simulink model "k1vissrmp_20190617"  (Simulink 8.6)
settings: Solver=ode45  StartTime=0.0  StopTime=10.0  RelTol=1e-3
libraries: cdsIPCx x5, cdsCDI64 x3, cdsCDO64 x3, TYPEB_MASTER x3, dac x2, cdsAdcx0 x1, cdsParameters x1
settings Model: Creator=controls  LastModifiedBy=controls
settings DataIOCC: SignalLoggingSaveFormat=Dataset
settings OptimizationCC: ExpressionDepthLimit=128
settings DebuggingCC: UnderspecifiedInitializationDetection=Simplified  MergeDetectMultiDrivingBlocksExec=error  SolverPrmCheckMsg=none  FcnCallInpInsideContextMsg=EnableAllAsError  StateNameClashWarn=none
settings GRTTargetCC: CombineOutputUpdateFcns=on  GRTInterface=off

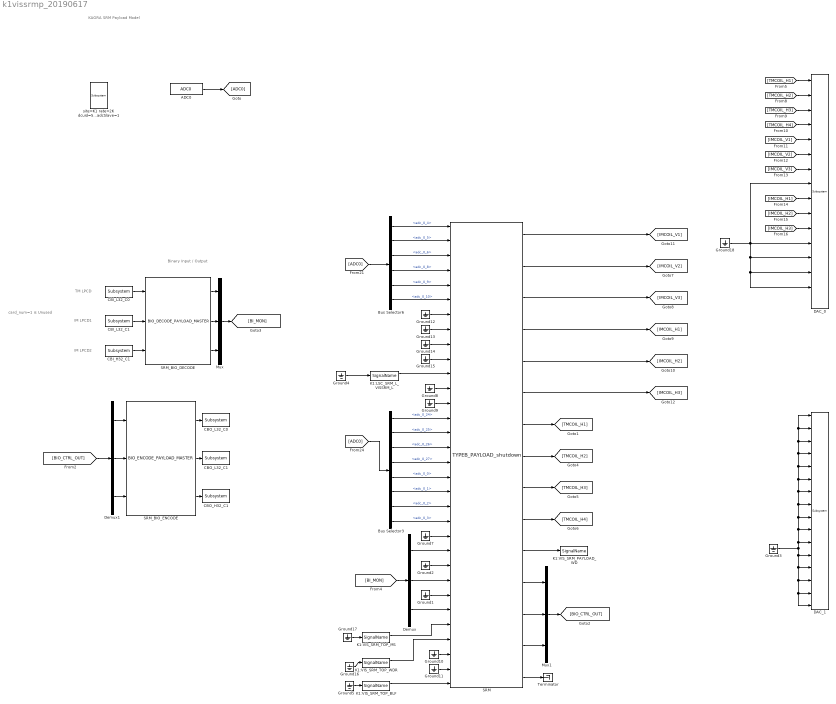
== system k1vissrmp_20190617 ==
  note: KAGRA SRM Payload Model
  note: Binary Input / Output
  note: TM LPCD
  note: card_num=1 is Unused
  note: IM LPCD1
  note: IM LPCD2
  ADC0 : cdsAdcx0/ADC0  Tag=cdsAdc  Description=|
      | type-GSC_16AI64SSA
      | card_num=0
      settings: AttributesFormatString=%<Description>\n%<Tag>
  Bus Selector3 : BusSelector  Description=ADC Selector  OutputSignals=adc_0_24,adc_0_25,adc_0_26,adc_0_27,adc_0_0,adc_0_1,adc_0_2,adc_0_3
      settings: AttributesFormatString=%<Description>
  Bus Selector6 : BusSelector  Description=ADC Selector  OutputSignals=adc_0_4,adc_0_5,adc_0_6,adc_0_8,adc_0_9,adc_0_10
      settings: AttributesFormatString=%<Description>
  CBI_H32_C1 : cdsCDI64/Subsystem  Tag=cdsCDI64  Description=card_num=3
      settings: AttributesFormatString=%<Tag>\n%<Description>
  CBI_L32_C0 : cdsCDI64/Subsystem  Tag=cdsCDI64  Description=card_num=0
      settings: AttributesFormatString=%<Tag>\n%<Description>
  CBI_L32_C1 : cdsCDI64/Subsystem  Tag=cdsCDI64  Description=card_num=2
      settings: AttributesFormatString=%<Tag>\n%<Description>
  CBO_H32_C1 : cdsCDO64/Subsystem  Tag=cdsCDO64  Description=card_num=3
      settings: AttributesFormatString=%<Tag>\n%<Description>
  CBO_L32_C0 : cdsCDO64/Subsystem  Tag=cdsCDO64  Description=card_num=0
      settings: AttributesFormatString=%<Tag>\n%<Description>
  CBO_L32_C1 : cdsCDO64/Subsystem  Tag=cdsCDO64  Description=card_num=2
      settings: AttributesFormatString=%<Tag>\n%<Description>
  DAC_0 : dac/Subsystem  Description=|
      | type=GSC_16AO16,
      | card_num=0
      settings: AttributesFormatString=%<Description>
  DAC_1 : dac/Subsystem  Description=|
      | type=GSC_16AO16,
      | card_num=1
      settings: AttributesFormatString=%<Description>
  Demux : Demux  Outputs=3
  Demux1 : Demux  Outputs=3
  Ground{1..5,7..18} (17 alike) : Ground
  K1:LSC_SRM_L_VISSRM_L : cdsIPCx/SignalName  Tag=cdsIPCx_PCIE  Description=Inter-Process Communication via PCI Express network.
      settings: AttributesFormatString=%<Tag>
  K1:VIS_SRM_PAYLOAD_WD : cdsIPCx/SignalName  Tag=cdsIPCx_SHMEM  Description=Inter-Process Communication via Shared memory.
      settings: AttributesFormatString=%<Tag>
  K1:VIS_SRM_TOP_BLF : cdsIPCx/SignalName  Tag=cdsIPCx_SHMEM  Description=Inter-Process Communication via Shared memory.
      settings: AttributesFormatString=%<Tag>
  K1:VIS_SRM_TOP_MS : cdsIPCx/SignalName  Tag=cdsIPCx_SHMEM  Description=Inter-Process Communication via Shared memory.
      settings: AttributesFormatString=%<Tag>
  K1:VIS_SRM_TOP_WDR : cdsIPCx/SignalName  Tag=cdsIPCx_SHMEM  Description=Inter-Process Communication via Shared memory.
      settings: AttributesFormatString=%<Tag>
  Mux : Mux  Inputs=3
  Mux1 : Mux  Inputs=3
  SRM : TYPEB_MASTER/TYPEB_PAYLOAD_shutdown
  SRM_BIO_DECODE : TYPEB_MASTER/BIO_DECODE_PAYLOAD_MASTER
  SRM_BIO_ENCODE : TYPEB_MASTER/BIO_ENCODE_PAYLOAD_MASTER
  Terminator : Terminator
  site=K1 rate=2K dcuid=59 host=k1srm specific_cpu=5 adcSlave=1 : cdsParameters/Subsystem  Tag=cdsParameters  Description=|
      | Purpose:                                                                                                                                                                                                                                
      | Provide system parameters to the FE code generator to properly configure the generated EPICS names, rep rate of the FE controller, and the Data Acquisition node ID for proper storage of data from this FE controller.                 
      |                                                                                                                                                                                                                                         
      | Useage:                                                                                                                                                                                                                                 
      | The part NAME field is used to identify the FE parameters. It must be of the form:                                                                                                                                                      
      | site=                                                                                                                                                                                                                                   
      | rate=                                                                                                                                                                                                                                   
      | dcuid=                                                                                                                                                                                                                                  
      |                                                                                                                                                                                                                                         
      | Where:                                                                                                                                                                                                                                  
      | site= argument may be H1, H2, L1, M1, G1, either as a single argument or multiple, for example site=H1,H2. These are the only names allowed. These will become the first two characters of all EPICS and signal names (for example G1:).
      |                                                                                                                                                                                                                                         
      | rate= may be 2K, 16K, 32K, or 64K                                                                                                                                                                                                       
      |                                                                                                                                                                                                                                         
      | dcuid= is site specific ie it must be unique at each site.
      settings: AttributesFormatString=%<Tag>
  wires:
  ADC0/1 -> [ADC0]
  [ADC0] -> Bus Selector6/1
  SRM/10 -> [TMCOIL_H4]
  SRM/9 -> [TMCOIL_H3]
  SRM/8 -> [TMCOIL_H2]
  SRM/7 -> [TMCOIL_H1]
  SRM/1 -> [IMCOIL_V1]
  SRM/2 -> [IMCOIL_V2]
  SRM/3 -> [IMCOIL_V3]
  SRM/4 -> [IMCOIL_H1]
  SRM/5 -> [IMCOIL_H2]
  SRM/6 -> [IMCOIL_H3]
  Ground18/1 -> DAC_0/12, DAC_0/13, DAC_0/14, DAC_0/15, DAC_0/8
  Bus Selector6/1 -> SRM/1  "<adc_0_4>"
  Bus Selector6/2 -> SRM/2  "<adc_0_5>"
  Bus Selector6/3 -> SRM/3  "<adc_0_6>"
  [TMCOIL_H2] -> DAC_0/2
  [TMCOIL_H3] -> DAC_0/3
  [TMCOIL_H1] -> DAC_0/1
  [TMCOIL_H4] -> DAC_0/4
  [IMCOIL_V1] -> DAC_0/5
  [IMCOIL_V2] -> DAC_0/6
  [IMCOIL_V3] -> DAC_0/7
  Bus Selector6/4 -> SRM/4  "<adc_0_8>"
  Bus Selector6/5 -> SRM/5  "<adc_0_9>"
  Bus Selector6/6 -> SRM/6  "<adc_0_10>"
  [IMCOIL_H3] -> DAC_0/11
  [IMCOIL_H2] -> DAC_0/10
  [IMCOIL_H1] -> DAC_0/9
  Ground8/1 -> SRM/12
  Ground9/1 -> SRM/13
  [ADC0] -> Bus Selector3/1
  Bus Selector3/1 -> SRM/14  "<adc_0_24>"
  Bus Selector3/2 -> SRM/15  "<adc_0_25>"
  Bus Selector3/3 -> SRM/16  "<adc_0_26>"
  Bus Selector3/4 -> SRM/17  "<adc_0_27>"
  SRM/11 -> K1:VIS_SRM_PAYLOAD_WD/1
  Mux1/1 -> [BIO_CTRL_OUT]
  SRM/13 -> Mux1/2
  [BI_MON] -> Demux/1
  Demux/1 -> SRM/23
  Demux/2 -> SRM/25
  Demux/3 -> SRM/27
  Ground7/1 -> SRM/22
  Ground1/1 -> SRM/26
  Ground2/1 -> SRM/24
  SRM/15 -> Terminator/1
  Ground3/1 -> DAC_1/13, DAC_1/14, DAC_1/15, DAC_1/16, DAC_1/12, DAC_1/7, DAC_1/6, DAC_1/5, DAC_1/1, DAC_1/2, DAC_1/3, DAC_1/4, DAC_1/8, DAC_1/9, DAC_1/10, DAC_1/11
  Bus Selector3/5 -> SRM/18  "<adc_0_0>"
  Bus Selector3/6 -> SRM/19  "<adc_0_1>"
  Bus Selector3/7 -> SRM/20  "<adc_0_2>"
  Bus Selector3/8 -> SRM/21  "<adc_0_3>"
  Ground12/1 -> SRM/7
  Ground13/1 -> SRM/8
  Ground14/1 -> SRM/9
  Ground15/1 -> SRM/10
  Ground10/1 -> SRM/30
  Ground11/1 -> SRM/31
  Ground16/1 -> K1:VIS_SRM_TOP_WDR/1
  Ground17/1 -> K1:VIS_SRM_TOP_MS/1
  K1:VIS_SRM_TOP_MS/1 -> SRM/28
  K1:VIS_SRM_TOP_WDR/1 -> SRM/29
  SRM_BIO_ENCODE/1 -> CBO_L32_C0/1
  SRM_BIO_ENCODE/3 -> CBO_H32_C1/1
  SRM_BIO_ENCODE/2 -> CBO_L32_C1/1
  CBI_L32_C1/1 -> SRM_BIO_DECODE/2
  CBI_H32_C1/1 -> SRM_BIO_DECODE/3
  SRM_BIO_DECODE/2 -> Mux/2
  SRM_BIO_DECODE/3 -> Mux/3
  SRM_BIO_DECODE/1 -> Mux/1
  Mux/1 -> [BI_MON]
  Demux1/2 -> SRM_BIO_ENCODE/2
  Demux1/3 -> SRM_BIO_ENCODE/3
  Demux1/1 -> SRM_BIO_ENCODE/1
  [BIO_CTRL_OUT] -> Demux1/1
  CBI_L32_C0/1 -> SRM_BIO_DECODE/1
  SRM/12 -> Mux1/1
  SRM/14 -> Mux1/3
  Ground5/1 -> K1:VIS_SRM_TOP_BLF/1
  K1:VIS_SRM_TOP_BLF/1 -> SRM/32
  Ground4/1 -> K1:LSC_SRM_L_VISSRM_L/1
  K1:LSC_SRM_L_VISSRM_L/1 -> SRM/11
